simulink model "inverted_pendulum"  (R2024b)
settings: Solver=ode1  StartTime=0.0  StopTime=100  FixedStep=1e-3  RelTol=1e-3
values from neighbouring files (symbols this model uses):
  Ac = [0 1;m*g*l/J (-b+K^2/R)/J]    [inverted_pendulum_script.m]
  Ad = [1, Ts; Ts*m*g*l/J, 1-Ts*(b+K^2/R)/J]    [inverted_pendulum_script.m]
  b = 3e-6    (= 3e-06)    [inverted_pendulum_script.m]
  Bc = [0; K/R/J]    [inverted_pendulum_script.m]
  Bd = [0; Ts*K/R/J]    [inverted_pendulum_script.m]
  Cd = [1, 0]    [inverted_pendulum_script.m]
  g = 9.81    [inverted_pendulum_script.m]
  J = 1.91e-4    (= 0.000191)    [inverted_pendulum_script.m]
  K = 0.0536    [inverted_pendulum_script.m]
  K_Gain = acker(Ac,Bc,p)    [inverted_pendulum_script.m]
  L = place(Ad', Cd', observer_poles)'    [inverted_pendulum_script.m]
  l = 0.042    [inverted_pendulum_script.m]
  m = 0.055    [inverted_pendulum_script.m]
  R = 9.5    [inverted_pendulum_script.m]
settings Model: Creator=costinchitic  LastModifiedBy=costinchitic

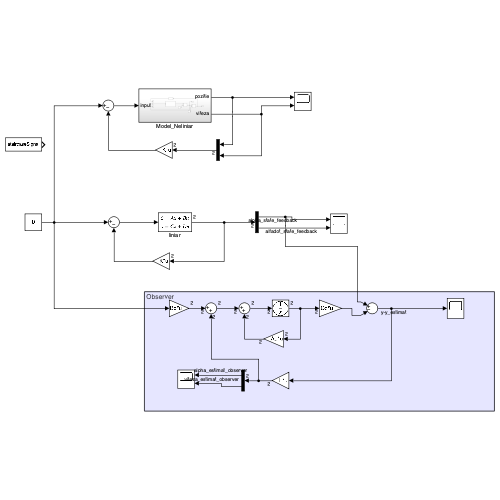
[thumbnail: Simulink's stored preview of the top-level diagram]
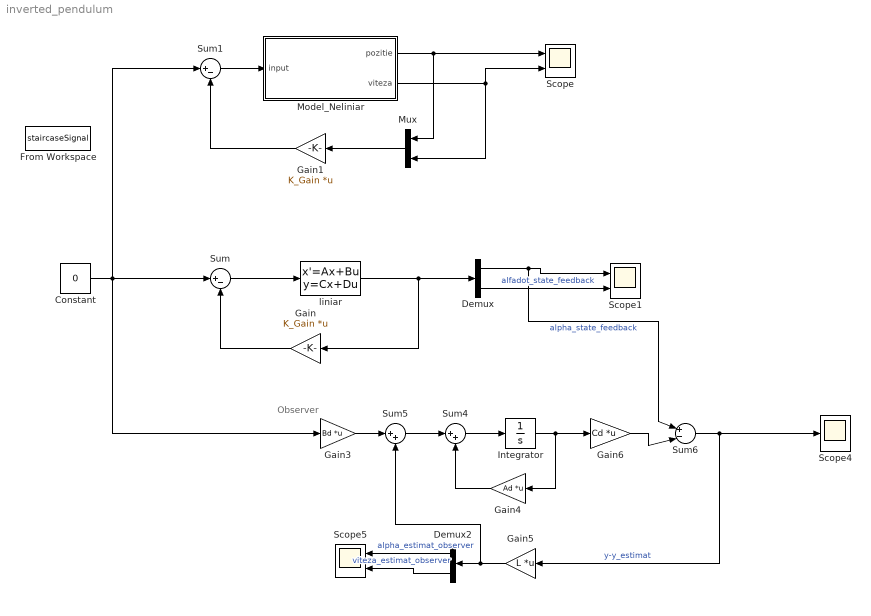
== system inverted_pendulum ==
  note: Observer
  Constant : Constant  Value=0
  Demux : Demux  Outputs=2
  Demux2 : Demux  Outputs=2
  From Workspace : FromWorkspace  VariableName=staircaseSignal
  Gain : Gain  Gain=K_Gain  Multiplication=Matrix(K*u)
  Gain1 : Gain  Gain=K_Gain  Multiplication=Matrix(K*u)
  Gain3 : Gain  Gain=Bd  Multiplication=Matrix(K*u)
  Gain4 : Gain  Gain=Ad  Multiplication=Matrix(K*u)
  Gain5 : Gain  Gain=L  Multiplication=Matrix(K*u)
  Gain6 : Gain  Gain=Cd  Multiplication=Matrix(K*u)
  Integrator : Integrator  InitialCondition=0.1  WrapState=on  WrappedStateUpperValue=2*pi  WrappedStateLowerValue=0
  Model_Neliniar : Subsystem
  Mux : Mux  Inputs=2
  Scope : Scope  NumInputPorts=2
  Scope1 : Scope  NumInputPorts=2
  Scope4 : Scope
  Scope5 : Scope  NumInputPorts=2
  Sum : Sum  Inputs=|+-
  Sum1 : Sum  Inputs=|+-
  Sum4 : Sum  Inputs=|++
  Sum5 : Sum  Inputs=|++
  Sum6 : Sum  Inputs=|+-|
  liniar : StateSpace  A=Ac  B=Bc  C=[1 0;0 1]  D=[0;0]  InitialCondition=[0.1 0]
  wires:
  Constant/1 -> Gain3/1, Sum1/1, Sum/1
  Gain/1 -> Sum/2
  Sum/1 -> liniar/1
  liniar/1 -> Demux/1, Gain/1
  Model_Neliniar/1(pozitie) -> Mux/1, Scope/1
  Model_Neliniar/2(viteza) -> Scope/2, Mux/2
  Mux/1 -> Gain1/1
  Gain1/1 -> Sum1/2
  Sum1/1 -> Model_Neliniar/1(input)
  Demux/1 -> Sum6/1, Scope1/1  "alpha_state_feedback"
  Demux/2 -> Scope1/2  "alfadot_state_feedback"
  Sum4/1 -> Integrator/1
  Gain4/1 -> Sum4/2
  Sum5/1 -> Sum4/1
  Gain3/1 -> Sum5/1
  Integrator/1 -> Gain4/1, Gain6/1
  Gain6/1 -> Sum6/2
  Sum6/1 -> Scope4/1, Gain5/1  "y-y_estimat"
  Gain5/1 -> Demux2/1, Sum5/2
  Demux2/1 -> Scope5/1  "alpha_estimat_observer"
  Demux2/2 -> Scope5/2  "viteza_estimat_observer"

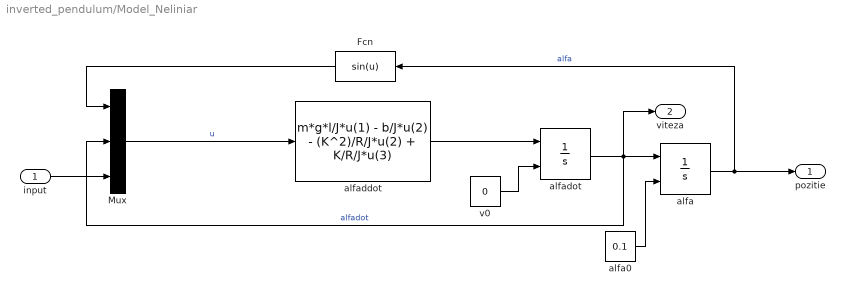
== system inverted_pendulum/Model_Neliniar ==
  input : Inport
  Fcn : Fcn  Expr=sin(u)
  Mux : Mux  Inputs=3
  alfa : Integrator  InitialConditionSource=external  WrapState=on  WrappedStateUpperValue=2*pi  WrappedStateLowerValue=0
  alfa0 : Constant  Value=0.1
  alfaddot : Fcn  Expr=m*g*l/J*u(1) - b/J*u(2) - (K^2)/R/J*u(2) + K/R/J*u(3)
  alfadot : Integrator  InitialConditionSource=external
  v0 : Constant  Value=0
  pozitie : Outport
  viteza : Outport  Port=2
  wires:
  v0/1 -> alfadot/2
  Mux/1 -> alfaddot/1  "u"
  input/1 -> Mux/3
  alfaddot/1 -> alfadot/1
  alfa/1 -> pozitie/1, Fcn/1  "alfa"
  alfa0/1 -> alfa/2
  alfadot/1 -> viteza/1, alfa/1, Mux/2  "alfadot"
  Fcn/1 -> Mux/1
